simulink model "Laba3"  (R2020b)
settings: Solver=VariableStepAuto  StartTime=0.0  StopTime=30  RelTol=1e-3
libraries: simulink x1
settings Model: Creator=ilya-  LastModifiedBy=Le tueur

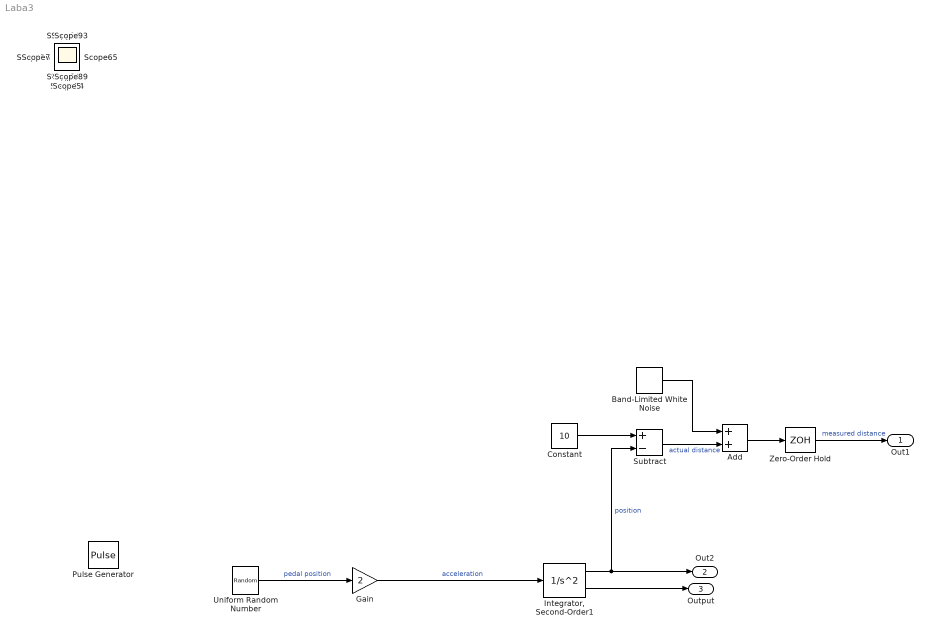
== system Laba3 ==
  Add : Sum
  Band-Limited White Noise : simulink/Sources/Band-Limited White Noise  Cov=0.001  Ts=0.1  seed=[23341]
  Constant : Constant  Value=10
  Gain : Gain  Gain=2
  "Integrator, Second-Order1" : SecondOrderIntegrator  LimitX=on  UpperLimitX=10
  Pulse Generator : DiscretePulseGenerator  PulseType=Time based  Period=10  PulseWidth=5
  Subtract : Sum  Inputs=+-
  Uniform Random Number : UniformRandomNumber  Minimum=0  SampleTime=0.1
  Zero-Order Hold : ZeroOrderHold  SampleTime=0.1
  Out1 : Outport
  Out2 : Outport  Port=2
  Output : Outport  Port=3
  Scope{,1..26} (27 alike) : Scope
  wires:
  Band-Limited White Noise/1 -> Add/1
  Constant/1 -> Subtract/1
  Add/1 -> Zero-Order Hold/1
  Zero-Order Hold/1 -> Out1/1  "measured distance"
  "Integrator, Second-Order1"/2 -> Output/1
  Gain/1 -> "Integrator, Second-Order1"/1  "acceleration"
  "Integrator, Second-Order1"/1 -> Subtract/2, Out2/1  "position"
  Subtract/1 -> Add/2  "actual distance"
  Uniform Random Number/1 -> Gain/1  "pedal position"
